simulink model "Simulink_6gdl_in_s"  (Simulink 7.8)
settings: Solver=ode45  StartTime=0.0  StopTime=10  FixedStep=10  MaxStep=0.01  MinStep=0.001  RelTol=1e-3
values from neighbouring files (symbols this model uses):
  Ad = inv(P)*A*M    [Matlab_6gdl_in_s.m]    (also in dimensionalizzazione ss.m)
  Bd = inv(P)*B    [Matlab_6gdl_in_s.m]    (also in dimensionalizzazione ss.m)
  C = eye(8)    [Matlab_6gdl_in_s.m]
  Cldelta = -Clp/80*2.2    (= 1.4575)    [Matlab_6gdl_in_s.m]
  Clp = -53    [Matlab_6gdl_in_s.m]
  D = zeros(8,1)    [Matlab_6gdl_in_s.m]
  diam = 0.079    [Matlab_6gdl_in_s.m]
  Ixap = Ixa * AR    (= 12878.3432699)    [Matlab_6gdl_in_s.m]
  Ve = 100    [Matlab_6gdl_in_s.m]
libraries: simulink x1
settings Model: Creator=Adriano  LastModifiedBy=Adriano
settings DataIOCC: LimitDataPoints=off  MaxDataPoints=5000

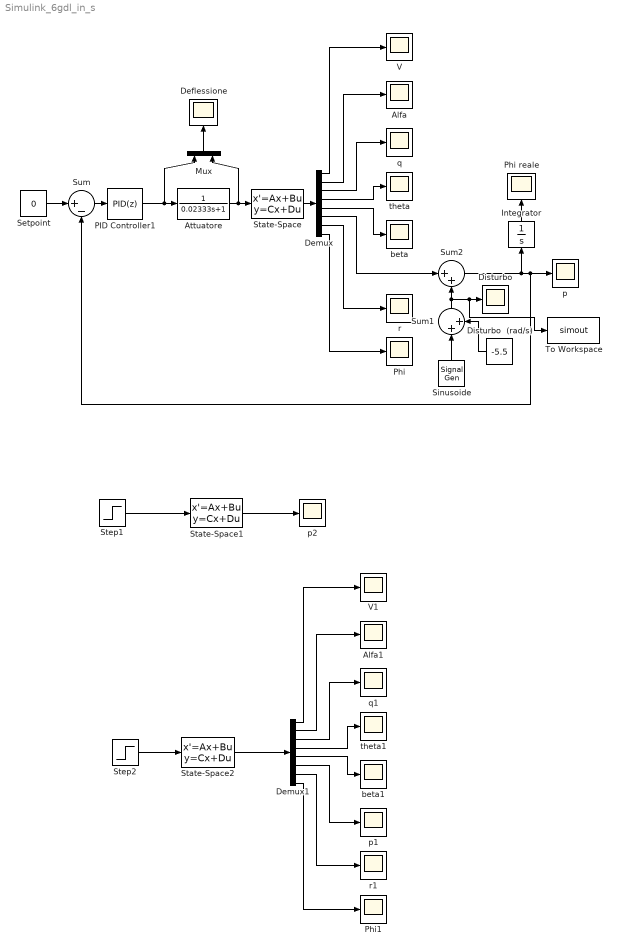
== system Simulink_6gdl_in_s ==
  Alfa : Scope
  Alfa1 : Scope
      settings: SaveName=ScopeData12
  Attuatore : TransferFcn  Denominator=[0.02333 1]
  Deflessione : Scope
      settings: SaveName=ScopeData10
  Demux : Demux  Outputs=8
  Demux1 : Demux  Outputs=8
  Disturbo : Scope
      settings: TimeRange=10  YMin=-6  YMax=-5  SaveName=ScopeData9
  Disturbo  (rad/s) : Constant  Value=-5.5
  Integrator : Integrator
  Mux : Mux  Inputs=2
  PID Controller1 : simulink/Continuous/PID Controller  Controller=PID  TimeDomain=Discrete-time  SampleTime=0.02  IntegratorMethod=Forward Euler  FilterMethod=Forward Euler  Form=Parallel  P=0.07  I=0.3  D=0.0233  N=1  InitialConditionSource=internal  InitialConditionForIntegrator=0  InitialConditionForFilter=0  ExternalReset=none  LimitOutput=on  UpperSaturationLimit=0.175  LowerSaturationLimit=-0.175  LinearizeAsGain=off  AntiWindupMode=clamping  Kb=1  TrackingMode=off  Kt=1  PParamMin=[]  PParamMax=[]  IParamMin=[]  IParamMax=[]  DParamMin=[]  DParamMax=[]  NParamMin=[]  NParamMax=[]  KbParamMin=[]  KbParamMax=[]  KtParamMin=[]  KtParamMax=[]  POutMin=[]  POutMax=[]  IOutMin=[]  IOutMax=[]  DOutMin=[]  DOutMax=[]  NOutMin=[]  NOutMax=[]  KbOutMin=[]  KbOutMax=[]  KtOutMin=[]  KtOutMax=[]  IntegratorOutMin=[]  IntegratorOutMax=[]  FilterOutMin=[]  FilterOutMax=[]  SumOutMin=[]  SumOutMax=[]  SumI1OutMin=[]  SumI1OutMax=[]  SumI2OutMin=[]  SumI2OutMax=[]  SumI3OutMin=[]  SumI3OutMax=[]  SumDOutMin=[]  SumDOutMax=[]  SaturationOutMin=[]  SaturationOutMax=[]  SaturationOutDataTypeStr=Inherit: Inherit via back propagation  IntegratorContinuousStateAttributes=''  IntegratorStateMustResolveToSignalObject=off  IntegratorRTWStateStorageClass=Auto  FilterContinuousStateAttributes=''  FilterStateMustResolveToSignalObject=off  FilterRTWStateStorageClass=Auto
  Phi : Scope
      settings: SaveName=ScopeData7
  Phi reale : Scope
      settings: SaveName=ScopeData11
  Phi1 : Scope
      settings: SaveName=ScopeData15
  Setpoint : Constant  Value=0
  Sinusoide : SignalGenerator  Amplitude=0.1  Frequency=2
  State-Space : StateSpace  A=Ad  B=Bd  C=C  D=D  X0=[0;0;0;0;0;0;0;0]  ContinuousStateAttributes='Variabili_di_stato'
  State-Space1 : StateSpace  A=(Clp/Ixap)*(2*Ve/diam)  B=(Cldelta/Ixap)*(2*Ve/diam)^2  D=0  ContinuousStateAttributes='Variabili_di_stato'
  State-Space2 : StateSpace  A=Ad  B=Bd  C=C  D=D  X0=[0;0;0;0;0;0;0;0]  ContinuousStateAttributes='Variabili_di_stato'
  Step1 : Step  After=0.17  SampleTime=0
  Step2 : Step  After=0.17  SampleTime=0
  Sum : Sum  Inputs=|+-
  Sum1 : Sum  Inputs=|++
  Sum2 : Sum  Inputs=|++
  To Workspace : ToWorkspace  VariableName=simout  SampleTime=-1  SaveFormat=Structure With Time
  V : Scope
  V1 : Scope
      settings: SaveName=ScopeData16
  beta : Scope
      settings: TimeRange=50  YMin=-0.01  YMax=0.06000000000000001  SaveName=ScopeData4
  beta1 : Scope
      settings: TimeRange=50  YMin=-0.01  YMax=0.06000000000000001  SaveName=ScopeData17
  p : Scope
      settings: SaveName=ScopeData5
  p1 : Scope
      settings: SaveName=ScopeData18
  p2 : Scope
      settings: SaveName=ScopeData8
  q : Scope
      settings: TimeRange=500  YMin=-1  YMax=1  SaveName=ScopeData2
  q1 : Scope
      settings: TimeRange=500  YMin=-1  YMax=1  SaveName=ScopeData19
  r : Scope
      settings: SaveName=ScopeData6
  r1 : Scope
      settings: SaveName=ScopeData20
  theta : Scope
      settings: SaveName=ScopeData3
  theta1 : Scope
      settings: SaveName=ScopeData21
  wires:
  Demux/1 -> V/1
  Demux/2 -> Alfa/1
  Demux/3 -> q/1
  Demux/4 -> theta/1
  Demux/5 -> beta/1
  Demux/7 -> r/1
  Demux/8 -> Phi/1
  Step1/1 -> State-Space1/1
  Setpoint/1 -> Sum/1
  State-Space/1 -> Demux/1
  State-Space1/1 -> p2/1
  PID Controller1/1 -> Mux/1, Attuatore/1
  Mux/1 -> Deflessione/1
  Attuatore/1 -> State-Space/1, Mux/2
  Sum/1 -> PID Controller1/1
  Disturbo  (rad/s)/1 -> Sum1/2
  Sinusoide/1 -> Sum1/1
  Sum1/1 -> Sum2/2, To Workspace/1, Disturbo/1
  Sum2/1 -> Sum/2, p/1, Integrator/1
  Demux/6 -> Sum2/1
  Integrator/1 -> Phi reale/1
  Demux1/1 -> V1/1
  Demux1/2 -> Alfa1/1
  Demux1/3 -> q1/1
  Demux1/4 -> theta1/1
  Demux1/5 -> beta1/1
  Demux1/7 -> r1/1
  Demux1/8 -> Phi1/1
  Demux1/6 -> p1/1
  State-Space2/1 -> Demux1/1
  Step2/1 -> State-Space2/1
